simulink model "FSAC2021_V1_Running"  (R2014a)
settings: Solver=FixedStepDiscrete  StartTime=0.0  StopTime=inf  FixedStep=0.0005  RelTol=1e-3
model workspace (MAT data in the model file):
  AS_READY = Simulink.Parameter
  AS_READY.Value = 2
  AS_READY.DataType = 'uint8'
  AS_DRIVING = Simulink.Parameter
  AS_DRIVING.Value = 3
  AS_DRIVING.DataType = 'uint8'
  AS_OFF = Simulink.Parameter
  AS_OFF.Value = 1
  AS_OFF.DataType = 'uint8'
  AS_FINISH = Simulink.Parameter
  AS_FINISH.Value = 4
  AS_FINISH.DataType = 'uint8'
  AS_EMERGENCY = Simulink.Parameter
  AS_EMERGENCY.Value = 5
  AS_EMERGENCY.DataType = 'uint8'
  ENABLE = Simulink.Parameter
  ENABLE.Value = 1
  ENABLE.DataType = 'uint8'
  DISABLE = Simulink.Parameter
  DISABLE.Value = 0
  DISABLE.DataType = 'uint8'
  Tire_Radius = Simulink.Parameter
  Tire_Radius.Value = 234
  Tire_Radius.DataType = 'single'
  Ts = Simulink.Parameter
  Ts.Value = 0.0005
  Ts.DataType = 'double'
  Filter_Factor = Simulink.Parameter
  Filter_Factor.Value = 0.5
  Filter_Factor.DataType = 'single'
  Teeth_Wheel = Simulink.Parameter
  Teeth_Wheel.Value = 60
  Teeth_Wheel.DataType = 'uint8'
  BLINK = Simulink.Parameter
  BLINK.Value = 2
  BLINK.DataType = 'uint8'
  OFF = Simulink.Parameter
  OFF.Value = 0
  OFF.DataType = 'uint8'
  ON = Simulink.Parameter
  ON.Value = 1
  ON.DataType = 'uint8'
  EBS_DISABLE = Simulink.Parameter
  EBS_DISABLE.Value = 0
  EBS_DISABLE.DataType = 'uint8'
  EBS_ARMED = Simulink.Parameter
  EBS_ARMED.Value = 1
  EBS_ARMED.DataType = 'uint8'
  EBS_ENABLE = Simulink.Parameter
  EBS_ENABLE.Value = 2
  EBS_ENABLE.DataType = 'uint8'
  MANUAL_DRIVING = Simulink.Parameter
  MANUAL_DRIVING.Value = 6
  MANUAL_DRIVING.DataType = 'uint8'
  MANUAL_MODE = Simulink.Parameter
  MANUAL_MODE.Value = 6
  MANUAL_MODE.DataType = 'uint8'
  BUZZER_START = 1
  BUZZER_EBS = Simulink.Parameter
  BUZZER_EBS.Value = 2
  BUZZER_EBS.DataType = 'uint8'
  TRACKDRIVE = Simulink.Parameter
  TRACKDRIVE.Value = 3
  TRACKDRIVE.DataType = 'uint8'
  Self_Learn_Diff = Simulink.Parameter
  Self_Learn_Diff.Value = 150
  Self_Learn_Diff.DataType = 'uint16'
  Acc_Left_Full_mv = Simulink.Parameter
  Acc_Left_Full_mv.Value = 2000
  Acc_Left_Full_mv.DataType = 'single'
  Acc_Right_Full_mv = Simulink.Parameter
  Acc_Right_Full_mv.Value = 2000
  Acc_Right_Full_mv.DataType = 'single'
  Brk_Calib_Value = Simulink.Parameter
  Brk_Calib_Value.Value = 150
  Brk_Calib_Value.DataType = 'single'
  Brk_Use_Range = Simulink.Parameter
  Brk_Use_Range.Value = 1500
  Brk_Use_Range.DataType = 'single'
  Armed = Simulink.Parameter
  Armed.Value = 1
  Armed.DataType = 'uint8'
  Enable = Simulink.Parameter
  Enable.Value = 2
  Enable.DataType = 'uint8'
  Disable = Simulink.Parameter
  Disable.Value = 0
  Disable.DataType = 'uint8'
  High_V = Simulink.Parameter
  High_V.Value = 60
  High_V.DataType = 'uint8'
  reg_num = Simulink.Parameter
  reg_num.Value = 1
  reg_num.DataType = 'uint8'
  Acc_Diff = Simulink.Parameter
  Acc_Diff.Value = 0.3
  Acc_Diff.DataType = 'single'
  Mtr_Cabli = Simulink.Parameter
  Mtr_Cabli.Value = 3
  Mtr_Cabli.DataType = 'single'
  BMS_Cabli = Simulink.Parameter
  BMS_Cabli.Value = 3
  BMS_Cabli.DataType = 'single'
  EBS_Cabli = Simulink.Parameter
  EBS_Cabli.Value = 3.3
  EBS_Cabli.DataType = 'single'
  Acc_Right_Factor = Simulink.Parameter
  Acc_Right_Factor.Value = -0.0833
  Acc_Right_Factor.DataType = 'double'
  Acc_Left_Factor = Simulink.Parameter
  Acc_Left_Factor.Value = 0.045
  Acc_Left_Factor.DataType = 'double'
  Acc_Lft_Offset = Simulink.Parameter
  Acc_Lft_Offset.Value = -90
  Acc_Lft_Offset.DataType = 'int8'
  Acc_Right_Offset = Simulink.Parameter
  Acc_Right_Offset.Value = 408.33
  Acc_Right_Offset.DataType = 'single'
  RTeeth_Wheel = Simulink.Parameter
  RTeeth_Wheel.Value = 30
  RTeeth_Wheel.DataType = 'uint8'
  FTeeth_Wheel = Simulink.Parameter
  FTeeth_Wheel.Value = 60
  FTeeth_Wheel.DataType = 'uint8'
  Brk_Liquid_Prs_Offset = Simulink.Parameter
  Brk_Liquid_Prs_Offset.Value = 0
  Brk_Liquid_Prs_Offset.DataType = 'single'
  Brk_Liquid_Prs_Factor = Simulink.Parameter
  Brk_Liquid_Prs_Factor.Value = 0.001
  Brk_Liquid_Prs_Factor.DataType = 'double'
  EBS_Prs_Factor = Simulink.Parameter
  EBS_Prs_Factor.Value = 0.000303
  EBS_Prs_Factor.DataType = 'double'
  EBS_Prs_Offset = Simulink.Parameter
  EBS_Prs_Offset.Value = 0
  EBS_Prs_Offset.DataType = 'single'
  Mtr_Volt_Factor = Simulink.Parameter
  Mtr_Volt_Factor.Value = 33.33
  Mtr_Volt_Factor.DataType = 'single'
  Mtr_Volt_Offset = Simulink.Parameter
  Mtr_Volt_Offset.Value = 0
  Mtr_Volt_Offset.DataType = 'single'
  BMS_Output_Volt_Factor = Simulink.Parameter
  BMS_Output_Volt_Factor.Value = 33.33
  BMS_Output_Volt_Factor.DataType = 'single'
  BMS_Output_Volt_Offset = Simulink.Parameter
  BMS_Output_Volt_Offset.Value = 0
  BMS_Output_Volt_Offset.DataType = 'single'
  Min = Simulink.Parameter
  Min.Value = 10
  Min.DataType = 'uint8'
  ACC_LOCK_UPSET = Simulink.Parameter
  ACC_LOCK_UPSET.Value = 25
  ACC_LOCK_UPSET.DataType = 'uint8'
  BRK_DISPSENS_LOWLIMIT = Simulink.Parameter
  BRK_DISPSENS_LOWLIMIT.Value = 2
  BRK_DISPSENS_LOWLIMIT.DataType = 'single'
  BRK_ENGAGED = Simulink.Parameter
  BRK_ENGAGED.Value = 1
  BRK_ENGAGED.DataType = 'uint8'
  BRK_Engaged_Angle = Simulink.Parameter
  BRK_Engaged_Angle.Value = 10
  BRK_Engaged_Angle.DataType = 'int8'
  BRK_MOVE = Simulink.Parameter
  BRK_MOVE.Value = 3
  BRK_MOVE.DataType = 'uint8'
  BRK_MTR_RATIO = Simulink.Parameter
  BRK_MTR_RATIO.Value = 10
  BRK_MTR_RATIO.DataType = 'uint8'
  BRK_TOZERO = Simulink.Parameter
  BRK_TOZERO.Value = 2
  BRK_TOZERO.DataType = 'uint8'
  Brake = 11
  Brk_Pct2Angle = Simulink.Parameter
  Brk_Pct2Angle.Value = 0.9
  Brk_Pct2Angle.DataType = 'single'
  Brk_Prop2Angle = Simulink.Parameter
  Brk_Prop2Angle.Value = 1
  Brk_Prop2Angle.DataType = 'single'
  DIFF_RATIO = Simulink.Parameter
  DIFF_RATIO.Value = 5
  DIFF_RATIO.DataType = 'uint8'
  DISABLE1 = Simulink.Parameter
  DISABLE1.Value = 0
  DISABLE1.DataType = 'uint8'
  ENABLE1 = Simulink.Parameter
  ENABLE1.Value = 1
  ENABLE1.DataType = 'uint8'
  MANUAL_MODEL = Simulink.Parameter
  MANUAL_MODEL.Value = 6
  MANUAL_MODEL.DataType = 'uint8'
  PULSES_PER_CIRCLE = Simulink.Parameter
  PULSES_PER_CIRCLE.Value = 6400
  PULSES_PER_CIRCLE.DataType = 'auto'
  Pct2Kmh = Simulink.Parameter
  Pct2Kmh.Value = 0.2
  Pct2Kmh.DataType = 'double'
  Sensor_Acc_b = 101.85
  Sensor_Acc_k = -0.0185
  Str_Sen_Orig_Angle = -341
  TIRE_D = Simulink.Parameter
  TIRE_D.Value = 0.47
  TIRE_D.DataType = 'double'
  Tire_D = 0.47
  T = 0.05
libraries: simulink x402, ec55xxlib x134
(part 1 of 17)
settings Model: Creator=zxj  LastModifiedBy=zxj
settings OptimizationCC: InlineParams=on  InlineInvariantSignals=on  RollThreshold=9  StateBitsets=on  DataBitsets=on  UseTempVars=on  ZeroExternalMemoryAtStartup=off  ZeroInternalMemoryAtStartup=off  EfficientFloat2IntCast=on  OptimizeModelRefInitCode=on  LifeSpan=1
settings DebuggingCC: InheritedTsInSrcMsg=none  ParameterOverflowMsg=none
settings HardwareCC: ProdLargestAtomicInteger=Long  ProdLargestAtomicFloat=Double  ProdIntDivRoundTo=Zero  ProdEndianess=BigEndian  ProdHWDeviceType=Freescale MPC5500
settings RTWCC: SystemTargetFile=ec55xx.tlc  MakeCommand=make_rtw optimized_fixed_point=1  GenerateMakefile=off  TemplateMakefile=ec55xx_lcc.tmf  PostCodeGenCommand=ec55xx_pst_s2(buildInfo)  Description=Target for EC55XX  GenerateReport=on  ProcessScript=ec55xx_make_rtw_hook  IncludeHyperlinkInReport=on  LaunchReport=on
settings CodeAppCC: IgnoreCustomStorageClasses=off
settings STFCustomTargetCC: ModelReferenceCompliant=off  ConcurrentExecutionCompliant=off  IncludeMdlTerminateFcn=off  GeneratePreprocessorConditionals=Use local settings  CombineOutputUpdateFcns=on  SuppressErrorStatus=on  ERTCustomFileBanners=on  SupportContinuousTime=off  SupportNonInlinedSFcns=off  MATLABClassNameForMDSCustomization=Simulink.SoftwareTarget.ERTCustomization  GRTInterface=off  SystemTargetFile=ec55xx.tlc
settings ERTTargetCC: GenerateSampleERTMain=off  ModelReferenceCompliant=off  IncludeMdlTerminateFcn=off  SuppressErrorStatus=on  GenerateASAP2=on  ERTSrcFileBannerTemplate=ec55xx_code_template.cgt  ERTHdrFileBannerTemplate=ec55xx_code_template.cgt  ERTDataSrcFileTemplate=ec55xx_code_template.cgt  ERTDataHdrFileTemplate=ec55xx_code_template.cgt  ERTCustomFileTemplate=ec55xx_file_process.tlc

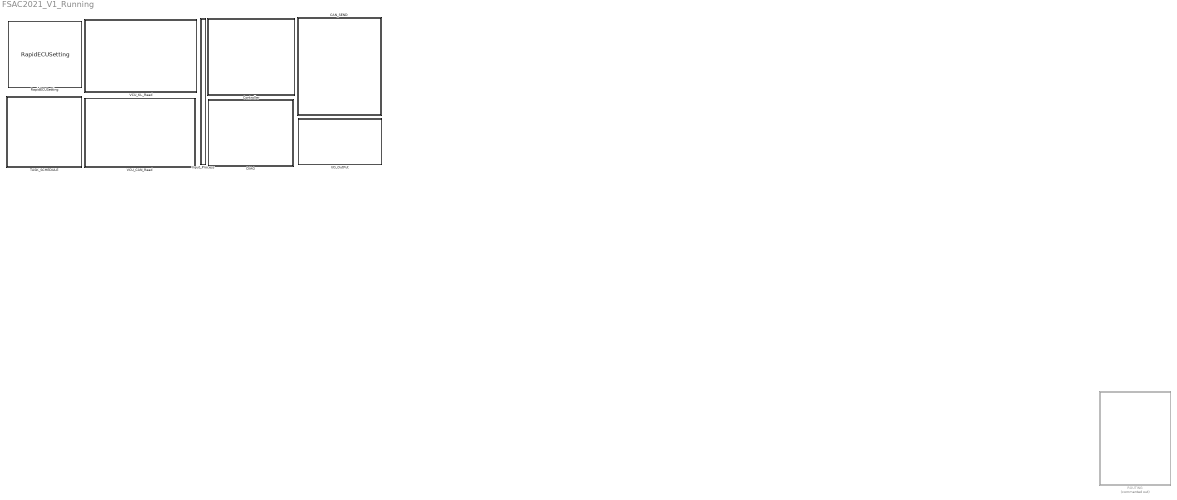
== system FSAC2021_V1_Running ==
  CAN_SEND : Subsystem
  Controller : Subsystem
  DIAG : Subsystem
  I/O_OutPut : Subsystem
  Input_Process : Subsystem
  ROUTING : Subsystem  Commented=on
  RapidECUSetting : ec55xxlib/RapidECU_U2/RapidECUSetting
      link override CAN: bcmt=Extended(29-bit ID)
      link override RTI: rtiperiod=0.0005
  TASK_SCHEDULE : Subsystem
  VCU_CAN_Read : Subsystem
  VCU_KL_Read : Subsystem

== system FSAC2021_V1_Running/CAN_SEND ==
  (BRK、STR、DRIVER) : Subsystem  SystemSampleTime=0.05
  From21 : From  Commented=on  GotoTag=Brk_Mtr_Enable_funCall  TagVisibility=global
  Rate Transition{1..19} (19 alike) : RateTransition  Deterministic=off
  Subsystem : Subsystem
  Subsystem1 : Subsystem
  Unit Delay{1..6} (6 alike) : UnitDelay  SampleTime=-1
  wires:
  [enable_operation_ctrl] -> Rate Transition4/1
  [new_set_pint_ctrl] -> Rate Transition5/1
  [abs_or_rel_ctrl] -> Rate Transition6/1
  [halt_ctrl] -> Rate Transition8/1
  [quick_stop_ctrl] -> Rate Transition3/1
  [enable_voltage_ctrl] -> Rate Transition2/1
  [position_set] -> Rate Transition9/1
  [switch_on_ctrl] -> Rate Transition1/1
  [nmt_nodeorder] -> Rate Transition11/1
  [nmt_nodectrl] -> Rate Transition12/1
  [encoder_msg_data] -> Rate Transition15/1
  [Brk_Mtr_GoalPos] -> Rate Transition17/1
  [Acc_Ctr] -> Rate Transition18/1
  Rate Transition17/1 -> Unit Delay3/1
  Rate Transition18/1 -> Unit Delay4/1
  Rate Transition10/1 -> Unit Delay5/1
  [BatVoltage_Out] -> Rate Transition10/1
  Rate Transition13/1 -> Unit Delay1/1
  Rate Transition14/1 -> Unit Delay2/1
  [Motor_Current_Speed] -> Rate Transition13/1
  [ASSI_State] -> Rate Transition14/1
  [Vel_Spd] -> Rate Transition16/1
  Rate Transition16/1 -> Unit Delay6/1
  [Fault_Reset] -> Rate Transition7/1
  Rate Transition7/1 -> Subsystem1/15(Fault_Reset)
  Rate Transition15/1 -> Subsystem1/14(Encoder_Msg_Data)
  [tmtsdocan] -> Subsystem1/13(Tmt_SDO_CAN_FunCall)
  [tmtnnmtcan] -> Subsystem1/10(Tmt_NMT_CAN_FunCall)
  Rate Transition11/1 -> Subsystem1/11(NMT_nodeorder)
  Rate Transition12/1 -> Subsystem1/12(NMT_nodectrl)
  [tmprdo1can] -> Subsystem1/1(Tmt_RPD01_CAN_FunCall)
  Rate Transition1/1 -> Subsystem1/2(Switch_On_Ctrl)
  Rate Transition6/1 -> Subsystem1/7(Abs_or_Rel_Ctrl)
  Rate Transition3/1 -> Subsystem1/4(Quick_Stop_Ctrl)
  Rate Transition2/1 -> Subsystem1/3(Enable_Voltage_Ctrl)
  Rate Transition4/1 -> Subsystem1/5(Enable_Operation_Ctrl)
  Rate Transition5/1 -> Subsystem1/6(New_Set_Point_Ctrl)
  Rate Transition8/1 -> Subsystem1/8(Halt_Ctrl)
  Rate Transition9/1 -> Subsystem1/9(Position_set)
  Unit Delay4/1 -> (BRK、STR、DRIVER)/2(Acc_Cmd)
  Unit Delay1/1 -> (BRK、STR、DRIVER)/4(Motor_Current_Speed)
  Unit Delay2/1 -> (BRK、STR、DRIVER)/5(ASSI_State)
  Unit Delay3/1 -> (BRK、STR、DRIVER)/1(Brk_Mtr_GoalPos)
  Unit Delay5/1 -> (BRK、STR、DRIVER)/3(BatVoltage_Out)
  Unit Delay6/1 -> (BRK、STR、DRIVER)/6(vspd)
  [ASSI_State] -> Rate Transition19/1
  Rate Transition19/1 -> Subsystem1/16(ASSI_STATE)

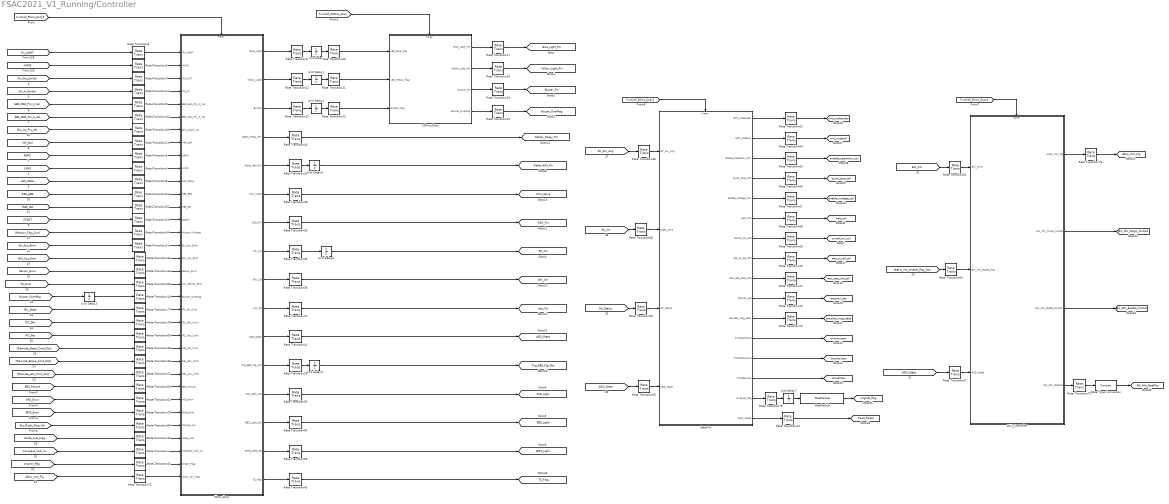
== system FSAC2021_V1_Running/Controller ==
  200ms_Duty : Subsystem
  50ms_Duty : Subsystem
  BCU_Controller : Subsystem
  Data Type Conversion : DataTypeConversion
  MeaModule : ec55xxlib/RapidECU_U2/11Calibration/MeaModule  signal=Steer_Origin_Flag
  Rate Transition{1..26,28..80} (79 alike) : RateTransition  Deterministic=off
  SteerCtr : Subsystem
  Unit Delay{,1..7} (8 alike) : UnitDelay  SampleTime=-1
  tag scope: ASSI_State=global, Acc_Ctr=global, Allow_Ctrl_Flg=global, BMS_Light=global, Blue_Light_Pin=global, Brk_Ctr=global, Brk_Mtr_Enable_funCall=global, Brk_Mtr_GoalPos=global, Brk_Mtr_Origin_funCall=global, Buzzer_Overflag=global, Buzzer_Pin=global, EBS_Light=global, Fault_Reset=global, IMD_Light=global, R2D_Pin=global, Relay_48V_Pin=global, Safety_Relay_Pin=global, Str_Ctr=global, TS_Flag=global, Trig_EBS_Flg_Out=global, VCU_Valve=global, Yellow_Light_Pin=global, abs_or_rel_ctrl=global, enable_operation_ctrl=global, enable_voltage_ctrl=global, encoder_msg_data=global, halt_ctrl=global, new_set_pint_ctrl=global, nmt_nodectrl=global, nmt_nodeorder=global, original_flag=global, position_set=global, quick_stop_ctrl=global, switch_on_ctrl=global, tmprdo1can=global, tmtnnmtcan=global, tmtsdocan=global
  wires:
  [On_Out_Switch] -> Rate Transition7/1
  [ASMS] -> Rate Transition5/1
  [AMI_State] -> Rate Transition8/1
  [EBS_GAS_Prs_2_Val] -> Rate Transition10/1
  [EBS_GAS_Prs_1_Val] -> Rate Transition9/1
  [HVMS] -> Rate Transition3/1
  Rate Transition8/1 -> 50ms_Duty/11(AMI_State)
  Rate Transition4/1 -> 50ms_Duty/10(LVMS)
  [LVMS] -> Rate Transition4/1
  Rate Transition10/1 -> 50ms_Duty/6(EBS_GAS_Prs_2_Val)
  Rate Transition7/1 -> 50ms_Duty/3(ON_OUT)
  [HV_LIGHT] -> Rate Transition2/1
  Rate Transition3/1 -> 50ms_Duty/2(HVMS)
  Rate Transition11/1 -> 50ms_Duty/8(Veh_Spd)
  Rate Transition2/1 -> 50ms_Duty/1(HV_LIGHT)
  [Vel_Spd] -> Rate Transition11/1
  Rate Transition9/1 -> 50ms_Duty/5(EBS_GAS_Prs_1_Val)
  Rate Transition5/1 -> 50ms_Duty/9(ASMS)
  [FunCall_50ms_Duty5] -> 50ms_Duty/Trigger
  [FunCall_200ms_Duty] -> 200ms_Duty/Trigger
  Rate Transition6/1 -> Unit Delay/1
  Rate Transition12/1 -> Unit Delay1/1
  Rate Transition13/1 -> Unit Delay2/1
  50ms_Duty/1(Blue_Light) -> Rate Transition6/1
  50ms_Duty/2(Yellow_Light) -> Rate Transition12/1
  50ms_Duty/3(Buzzer) -> Rate Transition13/1
  Unit Delay3/1 -> Rate Transition16/1
  Unit Delay/1 -> Rate Transition20/1
  Unit Delay1/1 -> Rate Transition21/1
  Unit Delay2/1 -> Rate Transition22/1
  [On_In_Switch] -> Rate Transition14/1
  Rate Transition14/1 -> 50ms_Duty/4(ON_IN)
  Rate Transition16/1 -> 50ms_Duty/20(Buzzer_Overflag)
  200ms_Duty/1(Blue_Light_Pin) -> Rate Transition17/1
  200ms_Duty/2(Yellow_Light_Pin) -> Rate Transition18/1
  200ms_Duty/3(Buzzer_Pin) -> Rate Transition19/1
  Rate Transition17/1 -> [Blue_Light_Pin]
  Rate Transition18/1 -> [Yellow_Light_Pin]
  Rate Transition19/1 -> [Buzzer_Pin]
  Rate Transition20/1 -> 200ms_Duty/1(LED_Blue_Flag)
  Rate Transition21/1 -> 200ms_Duty/2(LED_Yellow_Flag)
  Rate Transition22/1 -> 200ms_Duty/3(Buzzer_Flag)
  [START] -> Rate Transition23/1
  Rate Transition23/1 -> 50ms_Duty/14(START)
  [RES_EBS] -> Rate Transition24/1
  Rate Transition24/1 -> 50ms_Duty/12(RES_EBS)
  [RES_GO] -> Rate Transition25/1
  Rate Transition25/1 -> 50ms_Duty/13(RES_GO)
  Rate Transition26/1 -> 50ms_Duty/7(Brk_Liquid_Val)
  [Brs_Liq_Prs_Val] -> Rate Transition26/1
  200ms_Duty/4(Buzzer_Overflag) -> Rate Transition15/1
  Rate Transition15/1 -> [Buzzer_Overflag]
  [Buzzer_Overflag] -> Unit Delay3/1
  [Str_Sys_Error] -> Rate Transition31/1
  [Brk_Sys_Error] -> Rate Transition32/1
  [Sensor_Error] -> Rate Transition33/1
  Rate Transition31/1 -> 50ms_Duty/16(Str_Sys_Error)
  Rate Transition32/1 -> 50ms_Duty/17(Brk_Sys_Error)
  Rate Transition33/1 -> 50ms_Duty/18(Sensor_Error)
  [Mission_Flag_Out] -> Rate Transition34/1
  Rate Transition34/1 -> 50ms_Duty/15(Misson_Finished)
  50ms_Duty/8(Str_Ctr) -> Rate Transition35/1
  50ms_Duty/9(Brk_Ctr) -> Rate Transition36/1
  50ms_Duty/10(Acc_Ctr) -> Rate Transition37/1
  Rate Transition35/1 -> Unit Delay6/1
  Rate Transition36/1 -> [Brk_Ctr]
  Rate Transition37/1 -> [Acc_Ctr]
  Rate Transition38/1 -> [VCU_Valve]
  50ms_Duty/6(VCU_Valve) -> Rate Transition38/1
  Rate Transition39/1 -> [R2D_Pin]
  50ms_Duty/7(R2D_Pin) -> Rate Transition39/1
  50ms_Duty/4(Safety_Relay_Pin) -> Rate Transition40/1
  Rate Transition40/1 -> [Safety_Relay_Pin]
  50ms_Duty/11(ASSI_State) -> Rate Transition41/1
  Rate Transition41/1 -> [ASSI_State]
  [Node_Lost_Flag] -> Rate Transition42/1
  Rate Transition42/1 -> 50ms_Duty/31(Node_Lost)
  [Remote_Acc_Cmd_Out] -> Rate Transition47/1
  [Remote_Steer_Cmd_Out] -> Rate Transition49/1
  Rate Transition47/1 -> 50ms_Duty/26(Res_Acc_Cmd)
  [Remote_Brake_Cmd_Out] -> Rate Transition48/1
  Rate Transition49/1 -> 50ms_Duty/24(Res_Str_Cmd)
  Rate Transition48/1 -> 50ms_Duty/25(Res_Brk_Cmd)
  50ms_Duty/5(Relay_48V_Pin) -> Rate Transition30/1
  Rate Transition30/1 -> Unit Delay4/1
  Unit Delay4/1 -> [Relay_48V_Pin]
  [TS_Error] -> Rate Transition50/1
  Rate Transition50/1 -> 50ms_Duty/19(Acc_Sensor_Error)
  50ms_Duty/12(Trig_EBS_Flg_Out) -> Rate Transition28/1
  [EBS_Failure] -> Rate Transition51/1
  Rate Transition51/1 -> 50ms_Duty/27(EBS_Failure)
  Rate Transition28/1 -> Unit Delay5/1
  Unit Delay5/1 -> [Trig_EBS_Flg_Out]
  [BMS_Error] -> Rate Transition29/1
  Rate Transition29/1 -> 50ms_Duty/29(BMS_Error)
  Rate Transition52/1 -> 50ms_Duty/28(IMD_Error)
  [IMD_Error] -> Rate Transition52/1
  50ms_Duty/13(IMD_Light_Sts) -> Rate Transition53/1
  50ms_Duty/14(EBS_Light_Sts) -> Rate Transition54/1
  50ms_Duty/15(BMS_Light_Sts) -> Rate Transition55/1
  Rate Transition53/1 -> [IMD_Light]
  Rate Transition54/1 -> [EBS_Light]
  Rate Transition55/1 -> [BMS_Light]
  Rate Transition56/1 -> 50ms_Duty/30(Manual_Acc)
  [Acc_Right_Disp_Val] -> Rate Transition56/1
  SteerCtr/9(New_Set_Point_Ctrl) -> Rate Transition72/1
  SteerCtr/10(Position_set) -> Rate Transition73/1
  SteerCtr/11(Encoder_Msg_Data) -> Rate Transition74/1
  SteerCtr/2(NMT_nodectrl) -> Rate Transition64/1
  SteerCtr/3(Enable_Operation_Ctrl) -> Rate Transition65/1
  SteerCtr/4(Quick_Stop_Ctrl) -> Rate Transition66/1
  SteerCtr/5(Enable_Voltage_Ctrl) -> Rate Transition67/1
  SteerCtr/6(Halt_Ctrl) -> Rate Transition68/1
  SteerCtr/7(Switch_On_Ctrl) -> Rate Transition69/1
  SteerCtr/8(Abs_or_Rel_Ctrl) -> Rate Transition70/1
  SteerCtr/1(NMT_nodeorder) -> Rate Transition62/1
  [Str_Ctr] -> Rate Transition58/1
  [Str_Status] -> Rate Transition59/1
  [ASSI_State] -> Rate Transition60/1
  [Brk_Ctr] -> Rate Transition61/1
  [Brake_mtr_enable_flag_Out] -> Rate Transition63/1
  BCU_Controller/1(Allow_Ctrl_Flg) -> Rate Transition76/1
  BCU_Controller/4(Brk_Mtr_GoalPos) -> Rate Transition79/1
  Data Type Conversion/1 -> [Brk_Mtr_GoalPos]
  Rate Transition58/1 -> SteerCtr/2(Steer_Cmd)
  Rate Transition59/1 -> SteerCtr/3(Str_Status)
  Rate Transition60/1 -> SteerCtr/4(ASSI_State)
  Rate Transition61/1 -> BCU_Controller/1(Brk_Cmd)
  Rate Transition63/1 -> BCU_Controller/2(Brk_Mtr_Enable_Flg)
  Rate Transition62/1 -> [nmt_nodeorder]
  Rate Transition64/1 -> [nmt_nodectrl]
  Rate Transition65/1 -> [enable_operation_ctrl]
  Rate Transition66/1 -> [quick_stop_ctrl]
  Rate Transition67/1 -> [enable_voltage_ctrl]
  Rate Transition68/1 -> [halt_ctrl]
  Rate Transition69/1 -> [switch_on_ctrl]
  Rate Transition70/1 -> [abs_or_rel_ctrl]
  Rate Transition72/1 -> [new_set_pint_ctrl]
  Rate Transition73/1 -> [position_set]
  Rate Transition74/1 -> [encoder_msg_data]
  SteerCtr/15(Original_Flag) -> Rate Transition75/1
  Rate Transition76/1 -> [Allow_Ctrl_Flg]
  BCU_Controller/2(Brk_Mtr_Origin_funCall) -> [Brk_Mtr_Origin_funCall]
  BCU_Controller/3(Brk_Mtr_Enable_funCall) -> [Brk_Mtr_Enable_funCall]
  Rate Transition79/1 -> Data Type Conversion/1
  Rate Transition75/1 -> Unit Delay7/1
  SteerCtr/12(TmtNNMTCAN) -> [tmtnnmtcan]
  SteerCtr/13(TmtRPDO1CAN) -> [tmprdo1can]
  SteerCtr/14(TmtSDOCAN) -> [tmtsdocan]
  [FunCall_50ms_Duty1] -> SteerCtr/Trigger
  [FunCall_50ms_Duty3] -> BCU_Controller/Trigger
  Rate Transition1/1 -> 50ms_Duty/32(Compare_Volt_mv)
  [Compare_Volt_mv] -> Rate Transition1/1
  50ms_Duty/16(TS_Flag) -> Rate Transition43/1
  Rate Transition43/1 -> [TS_Flag]
  MeaModule/1 -> [original_flag]
  SteerCtr/16(Fault_Reset) -> Rate Transition44/1
  Rate Transition44/1 -> [Fault_Reset]
  Unit Delay6/1 -> [Str_Ctr]
  Rate Transition45/1 -> 50ms_Duty/33(Origin_Flag)
  [original_flag] -> Rate Transition45/1
  Unit Delay7/1 -> MeaModule/1
  [Str_Snr_Ang] -> Rate Transition46/1
  Rate Transition46/1 -> SteerCtr/1(Str_Snr_Ang)
  [ASSI_State] -> Rate Transition57/1
  Rate Transition57/1 -> BCU_Controller/3(ASSI_State)
  Rate Transition71/1 -> 50ms_Duty/34(Allow_Ctr_Flag)
  [Allow_Ctrl_Flg] -> Rate Transition71/1
  [IPC_Steer] -> Rate Transition77/1
  [IPC_Acc] -> Rate Transition80/1
  [IPC_Brk] -> Rate Transition78/1
  Rate Transition77/1 -> 50ms_Duty/21(IPC_Str_Cmd)
  Rate Transition78/1 -> 50ms_Duty/22(IPC_Brk_Cmd)
  Rate Transition80/1 -> 50ms_Duty/23(IPC_Acc_Cmd)

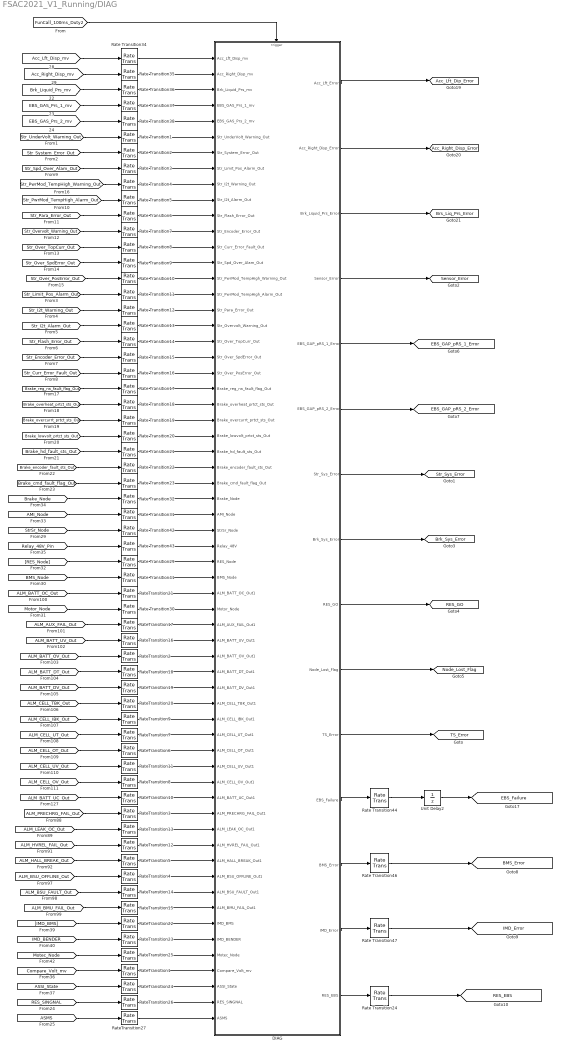
== system FSAC2021_V1_Running/DIAG ==
  DIAG : Subsystem
  Rate Transition{1..24,29..32,34..38,41..44,46..47} (39 alike) : RateTransition  Deterministic=off
  RateTransition{1..27} (27 alike) : RateTransition
  Unit Delay2 : UnitDelay  SampleTime=-1
  tag scope: Acc_Lft_Dip_Error=global, Acc_Right_Disp_Error=global, BMS_Error=global, Brk_Sys_Error=global, Brs_Liq_Prs_Error=global, EBS_Failure=global, EBS_GAP_pRS_1_Error=global, EBS_GAP_pRS_2_Error=global, IMD_Error=global, Node_Lost_Flag=global, RES_EBS=global, RES_GO=global, Sensor_Error=global, Str_Sys_Error=global, TS_Error=global
  wires:
  DIAG/1(Acc_Lft_Error) -> [Acc_Lft_Dip_Error]
  Rate Transition36/1 -> DIAG/3(Brk_Liquid_Prs_mv)
  DIAG/2(Acc_Right_Disp_Error) -> [Acc_Right_Disp_Error]
  DIAG/3(Brk_Liquid_Prs_Error) -> [Brs_Liq_Prs_Error]
  Rate Transition35/1 -> DIAG/2(Acc_Right_Disp_mv)
  Rate Transition37/1 -> DIAG/4(EBS_GAS_Prs_1_mv)
  Rate Transition38/1 -> DIAG/5(EBS_GAS_Prs_2_mv)
  Rate Transition34/1 -> DIAG/1(Acc_Lft_Disp_mv)
  [Brk_Liquid_Prs_mv] -> Rate Transition36/1
  [Acc_Lft_Disp_mv] -> Rate Transition34/1
  [EBS_GAS_Prs_1_mv] -> Rate Transition37/1
  [EBS_GAS_Prs_2_mv] -> Rate Transition38/1
  [Acc_Right_Disp_mv] -> Rate Transition35/1
  [FunCall_100ms_Duty2] -> DIAG/Trigger
  [Str_UnderVolt_Warning_Out] -> Rate Transition1/1
  [Str_System_Error_Out] -> Rate Transition2/1
  [Str_Spd_Over_Alam_Out] -> Rate Transition3/1
  [Str_PwrMod_TempHigh_Warning_Out] -> Rate Transition4/1
  [Str_PwrMod_TempHigh_Alarm_Out] -> Rate Transition5/1
  [Str_Para_Error_Out] -> Rate Transition6/1
  [Str_Overvolt_Warning_Out] -> Rate Transition7/1
  [Str_Over_TopCurr_Out] -> Rate Transition8/1
  [Str_Over_SpdError_Out] -> Rate Transition9/1
  [Str_Over_PosError_Out] -> Rate Transition10/1
  [Str_Limit_Pos_Alarm_Out] -> Rate Transition11/1
  [Str_I2t_Warning_Out] -> Rate Transition12/1
  [Str_I2t_Alarm_Out] -> Rate Transition13/1
  [Str_Flash_Error_Out] -> Rate Transition14/1
  [Str_Encoder_Error_Out] -> Rate Transition15/1
  [Str_Curr_Error_Fault_Out] -> Rate Transition16/1
  Rate Transition1/1 -> DIAG/6(Str_UnderVolt_Warning_Out)
  Rate Transition2/1 -> DIAG/7(Str_System_Error_Out)
  Rate Transition3/1 -> DIAG/8(Str_Limit_Pos_Alarm_Out)
  Rate Transition4/1 -> DIAG/9(Str_I2t_Warning_Out)
  Rate Transition5/1 -> DIAG/10(Str_I2t_Alarm_Out)
  Rate Transition6/1 -> DIAG/11(Str_Flash_Error_Out)
  Rate Transition7/1 -> DIAG/12(Str_Encoder_Error_Out)
  Rate Transition8/1 -> DIAG/13(Str_Curr_Error_Fault_Out)
  Rate Transition9/1 -> DIAG/14(Str_Spd_Over_Alam_Out)
  Rate Transition10/1 -> DIAG/15(Str_PwrMod_TempHigh_Warning_Out)
  Rate Transition11/1 -> DIAG/16(Str_PwrMod_TempHigh_Alarm_Out)
  Rate Transition12/1 -> DIAG/17(Str_Para_Error_Out)
  Rate Transition13/1 -> DIAG/18(Str_Overvolt_Warning_Out)
  Rate Transition15/1 -> DIAG/20(Str_Over_SpdError_Out)
  Rate Transition14/1 -> DIAG/19(Str_Over_TopCurr_Out)
  Rate Transition16/1 -> DIAG/21(Str_Over_PosError_Out)
  DIAG/4(Sensor_Error) -> [Sensor_Error]
  DIAG/7(Str_Sys_Error) -> [Str_Sys_Error]
  [Brake_overcurrt_prtct_sts_Out] -> Rate Transition19/1
  [Brake_overheat_prtct_sts_Out] -> Rate Transition18/1
  [Brake_reg_rw_fault_flag_Out] -> Rate Transition17/1
  [Brake_cmd_fault_flag_Out] -> Rate Transition23/1
  [Brake_hd_fault_sts_Out] -> Rate Transition21/1
  [Brake_encoder_fault_sts_Out] -> Rate Transition22/1
  [Brake_lowvolt_prtct_sts_Out] -> Rate Transition20/1
  Rate Transition17/1 -> DIAG/22(Brake_reg_rw_fault_flag_Out)
  Rate Transition18/1 -> DIAG/23(Brake_overheat_prtct_sts_Out)
  Rate Transition19/1 -> DIAG/24(Brake_overcurrt_prtct_sts_Out)
  Rate Transition20/1 -> DIAG/25(Brake_lowvolt_prtct_sts_Out)
  Rate Transition21/1 -> DIAG/26(Brake_hd_fault_sts_Out)
  Rate Transition22/1 -> DIAG/27(Brake_encoder_fault_sts_Out)
  Rate Transition23/1 -> DIAG/28(Brake_cmd_fault_flag_Out)
  DIAG/8(Brk_Sys_Error) -> [Brk_Sys_Error]
  DIAG/9(RES_GO) -> [RES_GO]
  [RES_Node] -> Rate Transition29/1
  [Motor_Node] -> Rate Transition30/1
  [AMI_Node] -> Rate Transition31/1
  [Brake_Node] -> Rate Transition32/1
  [BMS_Node] -> Rate Transition41/1
  [StrSr_Node] -> Rate Transition42/1
  Rate Transition29/1 -> DIAG/33(RES_Node)
  Rate Transition30/1 -> DIAG/36(Motor_Node)
  Rate Transition31/1 -> DIAG/30(AMI_Node)
  Rate Transition32/1 -> DIAG/29(Brake_Node)
  Rate Transition41/1 -> DIAG/34(BMS_Node)
  Rate Transition42/1 -> DIAG/31(StrSr_Node)
  DIAG/10(Node_Lost_Flag) -> [Node_Lost_Flag]
  [Relay_48V_Pin] -> Rate Transition43/1
  Rate Transition43/1 -> DIAG/32(Relay_48V)
  DIAG/11(TS_Error) -> [TS_Error]
  DIAG/5(EBS_GAP_pRS_1_Error) -> [EBS_GAP_pRS_1_Error]
  DIAG/12(EBS_Failure) -> Rate Transition44/1
  Rate Transition44/1 -> Unit Delay2/1
  Unit Delay2/1 -> [EBS_Failure]
  DIAG/6(EBS_GAP_pRS_2_Error) -> [EBS_GAP_pRS_2_Error]
  [ALM_BATT_OV_Out] -> RateTransition2/1
  RateTransition2/1 -> DIAG/39(ALM_BATT_OV_Out1)
  [ALM_PRECHRG_FAIL_Out] -> RateTransition3/1
  RateTransition3/1 -> DIAG/49(ALM_PRECHRG_FAIL_Out1)
  [ALM_BSU_OFFLINE_Out] -> RateTransition4/1
  RateTransition4/1 -> DIAG/53(ALM_BSU_OFFLINE_Out1)
  [ALM_HALL_BREAK_Out] -> RateTransition5/1
  RateTransition5/1 -> DIAG/52(ALM_HALL_BREAK_Out1)
  [ALM_CELL_OT_Out] -> RateTransition6/1
  RateTransition6/1 -> DIAG/45(ALM_CELL_OT_Out1)
  [ALM_CELL_UT_Out] -> RateTransition7/1
  RateTransition7/1 -> DIAG/44(ALM_CELL_UT_Out1)
  [ALM_CELL_OV_Out] -> RateTransition8/1
  RateTransition8/1 -> DIAG/47(ALM_CELL_OV_Out1)
  [ALM_CELL_IBK_Out] -> RateTransition9/1
  RateTransition9/1 -> DIAG/43(ALM_CELL_IBK_Out1)
  [ALM_BATT_UC_Out] -> RateTransition10/1
  RateTransition10/1 -> DIAG/48(ALM_BATT_UC_Out1)
  [ALM_CELL_UV_Out] -> RateTransition11/1
  RateTransition11/1 -> DIAG/46(ALM_CELL_UV_Out1)
  [ALM_HVREL_FAIL_Out] -> RateTransition12/1
  RateTransition12/1 -> DIAG/51(ALM_HVREL_FAIL_Out1)
  [ALM_LEAK_OC_Out] -> RateTransition13/1
  RateTransition13/1 -> DIAG/50(ALM_LEAK_OC_Out1)
  [ALM_BSU_FAULT_Out] -> RateTransition14/1
  RateTransition14/1 -> DIAG/54(ALM_BSU_FAULT_Out1)
  [ALM_BMU_FAIL_Out] -> RateTransition15/1
  RateTransition15/1 -> DIAG/55(ALM_BMU_FAIL_Out1)
  [ALM_BATT_UV_Out] -> RateTransition16/1
  RateTransition16/1 -> DIAG/38(ALM_BATT_UV_Out1)
  [ALM_AUX_FAIL_Out] -> RateTransition17/1
  RateTransition17/1 -> DIAG/37(ALM_AUX_FAIL_Out1)
  [ALM_BATT_DT_Out] -> RateTransition18/1
  RateTransition18/1 -> DIAG/40(ALM_BATT_DT_Out1)
  [ALM_BATT_DV_Out] -> RateTransition19/1
  RateTransition19/1 -> DIAG/41(ALM_BATT_DV_Out1)
  [ALM_CELL_TBK_Out] -> RateTransition20/1
  RateTransition20/1 -> DIAG/42(ALM_CELL_TBK_Out1)
  [ALM_BATT_OC_Out] -> RateTransition21/1
  RateTransition21/1 -> DIAG/35(ALM_BATT_OC_Out1)
  DIAG/13("BMS_Error ") -> Rate Transition46/1
  Rate Transition46/1 -> [BMS_Error]
  [IMD_BMS] -> RateTransition22/1
  [IMD_BENDER] -> RateTransition23/1
  RateTransition22/1 -> DIAG/56("IMD_BMS ")
  RateTransition23/1 -> DIAG/57("IMD_BENDER ")
  DIAG/14(IMD_Error) -> Rate Transition47/1
  Rate Transition47/1 -> [IMD_Error]
  RateTransition25/1 -> DIAG/58(Motec_Node)
  [Motec_Node] -> RateTransition25/1
  RateTransition1/1 -> DIAG/59(Compare_Volt_mv)
  [Compare_Volt_mv] -> RateTransition1/1
  RateTransition24/1 -> DIAG/60(ASSI_State)
  [ASSI_State] -> RateTransition24/1
  [RES_SINGNAL] -> RateTransition26/1
  RateTransition26/1 -> DIAG/61(RES_SINGNAL)
  [ASMS] -> RateTransition27/1
  RateTransition27/1 -> DIAG/62(ASMS)
  DIAG/15(RES_EBS) -> Rate Transition24/1
  Rate Transition24/1 -> [RES_EBS]

== system FSAC2021_V1_Running/I//O_OutPut ==
  Subsystem : Subsystem
  wires:
  [Blue_Light_Pin] -> Subsystem/1(Blue_Light_Pin)
  [Yellow_Light_Pin] -> Subsystem/2(Yellow_Light_Pin)
  [Buzzer_Pin] -> Subsystem/3(Buzzer_pin)
  [Safety_Relay_Pin] -> Subsystem/4(Safety_Relay_Pin)
  [Relay_48V_Pin] -> Subsystem/5(Relay_48V_Pin)
  [R2D_Pin] -> Subsystem/6(R2D_pin)
  [VCU_Valve] -> Subsystem/7(VCU_valve)
  [IMD_Light] -> Subsystem/8(IMD_Light)
  [EBS_Light] -> Subsystem/9(EBS_Light)
  [BMS_Light] -> Subsystem/10(BMS_Light)
  [FunCall_50ms_Duty10] -> Subsystem/Trigger

== system FSAC2021_V1_Running/Input_Process ==
  KL_Sig_Process : Subsystem
  Rate Transition{3..7,9..12,14..15,18..19,21..26} (19 alike) : RateTransition  Deterministic=off
  tag scope: Acc_Lft_Dip_Val=global, Acc_Right_Disp_Val=global, Brs_Liq_Prs_Val=global, EBS_GAS_Prs_1_Val=global, EBS_GAS_Prs_2_Val=global, Vel_Spd=global, Whl_Spd_FF_Val=global, Whl_Spd_FL_Val=global, Whl_Spd_RL_Val=global, Whl_Spd_RR_Val=global
  wires:
  [Acc_Lft_Disp_mv] -> Rate Transition21/1
  [EBS_GAS_Prs_1_mv] -> Rate Transition14/1
  [EBS_GAS_Prs_2_mv] -> Rate Transition24/1
  [Brk_Liquid_Prs_mv] -> Rate Transition23/1
  [Acc_Right_Disp_mv] -> Rate Transition22/1
  KL_Sig_Process/1(Vel_Spd) -> Rate Transition15/1
  KL_Sig_Process/4(Whl_Spd_RL_Val) -> Rate Transition10/1
  KL_Sig_Process/2(Whl_Spd_FL_Val) -> Rate Transition12/1
  KL_Sig_Process/3(Whl_Spd_FF_Val) -> Rate Transition11/1
  Rate Transition19/1 -> KL_Sig_Process/2(FR_WhlSpd_Hz)
  KL_Sig_Process/5(Whl_Spd_RR_Val) -> Rate Transition9/1
  Rate Transition26/1 -> KL_Sig_Process/4(RR_WhlSpd_Hz)
  [RR_WhlSpd_Hz] -> Rate Transition26/1
  Rate Transition25/1 -> KL_Sig_Process/3(RL_WhlSpd_Hz)
  Rate Transition18/1 -> KL_Sig_Process/1(FL_WhlSpd_Hz)
  [RL_WhlSpd_Hz] -> Rate Transition25/1
  [FL_WhlSpd_Hz] -> Rate Transition18/1
  [FR_WhlSpd_Hz] -> Rate Transition19/1
  KL_Sig_Process/7(Acc_Right_Disp_Val) -> Rate Transition6/1
  KL_Sig_Process/6(Acc_Lft_Disp_Val) -> Rate Transition7/1
  Rate Transition24/1 -> KL_Sig_Process/9(EBS_GAS_Prs_2_mv)
  Rate Transition23/1 -> KL_Sig_Process/7(Brk_Liquid_Prs_mv)
  KL_Sig_Process/10(EBS_GAS_Prs_2_Val) -> Rate Transition3/1
  Rate Transition21/1 -> KL_Sig_Process/5(Acc_Lft_Disp_mv)
  KL_Sig_Process/8(Brk_Liquid_Prs_Val) -> Rate Transition5/1
  Rate Transition22/1 -> KL_Sig_Process/6(Acc_Right_Disp_mv)
  KL_Sig_Process/9(EBS_GAS_Prs_1_Val) -> Rate Transition4/1
  Rate Transition14/1 -> KL_Sig_Process/8(EBS_GAS_Prs_1_mv)
  [FunCall_20ms_Duty] -> KL_Sig_Process/Trigger
  Rate Transition3/1 -> [EBS_GAS_Prs_2_Val]
  Rate Transition4/1 -> [EBS_GAS_Prs_1_Val]
  Rate Transition5/1 -> [Brs_Liq_Prs_Val]
  Rate Transition6/1 -> [Acc_Right_Disp_Val]
  Rate Transition7/1 -> [Acc_Lft_Dip_Val]
  Rate Transition9/1 -> [Whl_Spd_RR_Val]
  Rate Transition10/1 -> [Whl_Spd_RL_Val]
  Rate Transition11/1 -> [Whl_Spd_FF_Val]
  Rate Transition12/1 -> [Whl_Spd_FL_Val]
  Rate Transition15/1 -> [Vel_Spd]

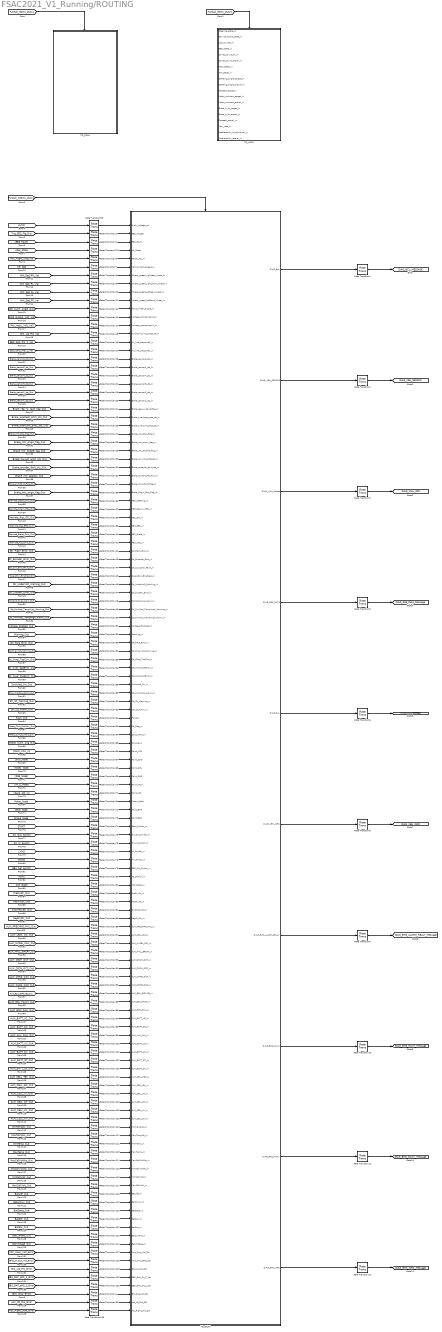
== system FSAC2021_V1_Running/ROUTING ==
  Rate Transition{1..4,6..130} (129 alike) : RateTransition  Deterministic=off
  Rate Transtion{1..3,5..6,8..12,33,131} (12 alike) : RateTransition  Deterministic=off
  TO_ACAN : Subsystem
  TO_DCAN : Subsystem
  TO_PCAN : Subsystem
  tag scope: DIAG_BCU_MESSAGE=global, DIAG_BMS_ALARM_RELAY_Message=global, DIAG_BMS_INFO_Message=global, DIAG_BMS_MAXT_Message=global, DIAG_BMS_MAXV_Message=global, DIAG_RES_Data_Message=global, DIAG_SCU_Message=global, DIAG_VEH_INFO=global, DIAG_VEH_SENSOR=global, DIAG_WHL_SPD=global
  wires:
  [FunCall_50ms_Duty4] -> TO_PCAN/Trigger
  [FunCall_50ms_Duty3] -> TO_ACAN/Trigger
  [Trig_EBS_Flg_Out] -> Rate Transition1/1
  [Whl_Spd_RL_Val] -> Rate Transition9/1
  [Brake_reg_rw_fault_flag_Out] -> Rate Transition24/1
  [BMS_Output_Volt_Val] -> Rate Transition13/1
  [Vel_Spd] -> Rate Transition7/1
  [Mtr_Input_Volt_Val] -> Rate Transition14/1
  [Brake_mtr_enable_flag_Out] -> Rate Transition29/1
  [EBS_GAS_Prs_1_Val] -> Rate Transition17/1
  [Brake_mtr_origin_flag_Out] -> Rate Transition28/1
  [Brake_encoder_fault_sts_Out] -> Rate Transition31/1
  [Whl_Spd_FL_Val] -> Rate Transition10/1
  [Brake_sensor5_sts_Out] -> Rate Transition20/1
  [Str_Currt_Angle_Out] -> Rate Transition12/1
  [EBS_Fault] -> Rate Transition2/1
  [Whl_Spd_FF_Val] -> Rate Transition11/1
  [Whl_Spd_RR_Val] -> Rate Transition8/1
  [Brake_overcurrt_prtct_sts_Out] -> Rate Transition26/1
  [Brake_lowvolt_prtct_sts_Out] -> Rate Transition30/1
  [Brake_sensor3_sts_Out] -> Rate Transition22/1
  [Str_Flash_Error_Out] -> Rate Transition42/1
  [Str_Over_PosError_Out] -> Rate Transition57/1
  [Str_Encoder_Error_Out] -> Rate Transition43/1
  [Motec_Currt_Current_Out] -> Rate Transition64/1
  [Str_PwrMod_TempHigh_Alarm_Out] -> Rate Transition50/1
  [Brake_mtr_stop_flag_Out] -> Rate Transition27/1
  [EBS_GAS_Prs_2_Val] -> Rate Transition16/1
  [Brake_mtr_goalpos_Out] -> Rate Transition32/1
  [Remote_Brake_Cmd_Out] -> Rate Transition40/1
  [Remote_Res_EBS_Out] -> Rate Transition38/1
  [Point_VCU_in] -> Rate Transition66/1
  [Brake_sensor1_sts_Out] -> Rate Transition23/1
  [Brake_sensor6_sts_Out] -> Rate Transition18/1
  [Str_Curr_Error_Fault_Out] -> Rate Transition44/1
  [Brake_sensor4_sts_Out] -> Rate Transition21/1
  [Str_System_Error_Out] -> Rate Transition47/1
  [Remote_Res_GO_Out] -> Rate Transition39/1
  [Fault_Out] -> Rate Transition62/1
  [Remote_Acc_Cmd_Out] -> Rate Transition41/1
  [Brs_Liq_Prs_Val] -> Rate Transition15/1
  [Operation_Enabled_Out] -> Rate Transition45/1
  [Remote_Steer_Cmd_Out] -> Rate Transition36/1
  [Remote_Origin_Flag_Out] -> Rate Transition37/1
  [Brake_sensor2_sts_Out] -> Rate Transition19/1
  [Brake_cmd_fault_flag_Out] -> Rate Transition34/1
  [Str_Spd_Over_Alam_Out] -> Rate Transition48/1
  [Str_I2t_Alarm_Out] -> Rate Transition61/1
  [Str_PwrMod_TempHigh_Warning_Out] -> Rate Transition49/1
  [Str_UnderVolt_Warning_Out] -> Rate Transition46/1
  [Str_Para_Error_Out] -> Rate Transition53/1
  [Voltage_Enabled_Out] -> Rate Transition51/1
  [Brake_mtr_origin_flag_Out] -> Rate Transition35/1
  [ALM_HALL_BREAK_Out] -> Rate Transition89/1
  [PreRlyStr_Out] -> Rate Transition82/1
  [MCU_Node] -> Rate Transition70/1
  [EBS_Rel_Switch] -> Rate Transition79/1
  [HVMS] -> Rate Transition78/1
  [ALM_CHRG_OCT_Out] -> Rate Transition92/1
  [StrSr_Node] -> Rate Transition67/1
  [RES_Node] -> Rate Transition69/1
  [ALM_CHRG_OCS_Out] -> Rate Transition93/1
  [OnChrRlyStr_Out] -> Rate Transition84/1
  [ALM_BMU_FAIL_Out] -> Rate Transition96/1
  [Motec_Node] -> Rate Transition68/1
  [Str_Over_SpdError_Out] -> Rate Transition56/1
  [PosRlyStr_Out] -> Rate Transition83/1
  [Point_IPC_in] -> Rate Transition71/1
  [ALM_DSCH_OCS_Out] -> Rate Transition91/1
  [BMS_Node] -> Rate Transition72/1
  [Str_Over_TopCurr_Out] -> Rate Transition55/1
  [Swtiched_On_Out] -> Rate Transition58/1
  [Str_I2t_Warning_Out] -> Rate Transition60/1
  [START] -> Rate Transition74/1
  [Str_Limit_Pos_Alarm_Out] -> Rate Transition59/1
  [AMI_State] -> Rate Transition81/1
  [Brake_Node] -> Rate Transition73/1
  [Str_Overvolt_Warning_Out] -> Rate Transition54/1
  [On_Out_Switch] -> Rate Transition75/1
  [On_In_Switch] -> Rate Transition76/1
  [ALM_PRECHRG_FAIL_Out] -> Rate Transition86/1
  [Warning_Out] -> Rate Transition52/1
  [LVMS] -> Rate Transition77/1
  [ASMS] -> Rate Transition80/1
  [ALM_BATT_OC_Out] -> Rate Transition98/1
  [ALM_CELL_TBK_Out] -> Rate Transition104/1
  [ALM_HVREL_FAIL_Out] -> Rate Transition88/1
  [ALM_BSU_OFFLINE_Out] -> Rate Transition94/1
  [ALM_CELL_OT_Out] -> Rate Transition107/1
  [MaxTempNo_Out] -> Rate Transition111/1
  [MinTemp_Out] -> Rate Transition112/1
  [ALM_BATT_DT_Out] -> Rate Transition102/1
  [ALM_LEAK_OC_Out] -> Rate Transition87/1
  [ALM_CELL_UT_Out] -> Rate Transition106/1
  [ALM_CELL_UV_Out] -> Rate Transition108/1
  [BatCurrent_Out] -> Rate Transition123/1
  [ALM_DSCH_OCT_Out] -> Rate Transition90/1
  [MaxTemp_Out] -> Rate Transition113/1
  [ALM_CELL_OV_Out] -> Rate Transition109/1
  Rate Transition1/1 -> TO_DCAN/2(EBS_Trigger)
  Rate Transition2/1 -> TO_DCAN/3(EBS_Fault)
  [ALM_CELL_IBK_Out] -> Rate Transition105/1
  [BatState_Out] -> Rate Transition120/1
  [MaxCellVolt_Out] -> Rate Transition117/1
  [ALM_BSU_FAULT_Out] -> Rate Transition95/1
  [MinTempNo_Out] -> Rate Transition110/1
  [ALM_BATT_DV_Out] -> Rate Transition103/1
  [BatSoc_Out] -> Rate Transition122/1
  [ALM_AUX_FAIL_Out] -> Rate Transition99/1
  [HVMS] -> Rate Transtion33/1
  [ALM_BATT_OV_Out] -> Rate Transition101/1
  [ASSI_State] -> Rate Transtion131/1
  [MinCellVoltNo_Out] -> Rate Transition115/1
  [ALM_BATT_UC_Out] -> Rate Transition97/1
  [ALM_BATT_UV_Out] -> Rate Transition100/1
  [NegRlyStr_Out] -> Rate Transition85/1
  [MaxCellVoltNo_Out] -> Rate Transition114/1
  Rate Transition11/1 -> TO_DCAN/10(Wheel_speed_leftfront_wheel_in)
  Rate Transition8/1 -> TO_DCAN/7(Wheel_speed_rightrear_whee_in)
  Rate Transition17/1 -> TO_DCAN/16(Air_line_pressure1_in)
  Rate Transition34/1 -> TO_DCAN/32(Brake_cmd_fault_flag_in)
  Rate Transition24/1 -> TO_DCAN/23(Brake_reg_rw_fault_flag_in)
  Rate Transition9/1 -> TO_DCAN/8(Wheel_speed_right_front_wheel_in)
  Rate Transition35/1 -> TO_DCAN/33(Brake_0rigin_End_flag_in)
  Rate Transition23/1 -> TO_DCAN/22(Brake_sensor1_sts_in)
  Rate Transition27/1 -> TO_DCAN/26(Brake_mtr_stop_flag_in)
  Rate Transition30/1 -> TO_DCAN/29(Brake_lowvolt_prtct_sts_in)
  [BatSoh_Out] -> Rate Transition121/1
  [BatVoltage_Out] -> Rate Transition124/1
  Rate Transition7/1 -> TO_DCAN/6(Veh_Current_Speed_in)
  Rate Transition14/1 -> TO_DCAN/13(Voltage_comparison1_in)
  Rate Transition26/1 -> TO_DCAN/25(Brake_overcurrt_prtct_sts_in)
  [Motec_Currt_Position_Out] -> Rate Transition63/1
  Rate Transition18/1 -> TO_DCAN/17(Brake_sensor6_sts_in)
  Rate Transition16/1 -> TO_DCAN/15(Air_line_pressure2_in)
  Rate Transition15/1 -> TO_DCAN/14(Hydraulic_line_pressure_in)
  Rate Transition20/1 -> TO_DCAN/18(Brake_sensor5_sts_in)
  Rate Transition6/1 -> TO_DCAN/5(Pedal_Acc_in)
  Rate Transition13/1 -> TO_DCAN/12(Voltage_comparison2_in)
  Rate Transition32/1 -> TO_DCAN/31(Brake_Current_Position_in)
  [Brake_overheat_prtct_sts_Out] -> Rate Transition25/1
  [BatAlmLv_Out] -> Rate Transition119/1
  [MinCellVolt_Out] -> Rate Transition116/1
  [BatLife_Out] -> Rate Transition118/1
  [Motec_Currt_Ang_Out] -> Rate Transition65/1
  Rate Transition12/1 -> TO_DCAN/11(Front_wheel_angle_in)
  Rate Transition10/1 -> TO_DCAN/9(Wheel_speed_leftrear_wheel_in)
  Rate Transition48/1 -> TO_DCAN/46(Str_Spd_Over_Alam_in)
  Rate Transition22/1 -> TO_DCAN/20(Brake_sensor3_sts_in)
  Rate Transition28/1 -> TO_DCAN/27(Brake_mtr_origin_flag_in)
  Rate Transition37/1 -> TO_DCAN/35(RES_Return_INFO_in)
  Rate Transition46/1 -> TO_DCAN/44(Str_UnderVolt_Warning_in)
  Rate Transition51/1 -> TO_DCAN/49(Voltage_Enabled_in)
  Rate Transition66/1 -> TO_DCAN/64(Point_VCU)
  Rate Transition40/1 -> TO_DCAN/38(RES_Brake_in)
  Rate Transition29/1 -> TO_DCAN/28(Brake_mtr_enable_flag_in)
  Rate Transition65/1 -> TO_DCAN/63(Str_Ang_in)
  Rate Transition41/1 -> TO_DCAN/39(RES_ACC_in)
  Rate Transition45/1 -> TO_DCAN/43(Operation_Enabled_in)
  Rate Transition44/1 -> TO_DCAN/42(Str_Curr_Error_Fault_in)
  Rate Transition62/1 -> TO_DCAN/60(Fault_in)
  Rate Transition21/1 -> TO_DCAN/19(Brake_sensor4_sts_in)
  Rate Transition42/1 -> TO_DCAN/40(Str_Flash_Error_in)
  Rate Transition53/1 -> TO_DCAN/51(Str_Para_Error_in)
  Rate Transition59/1 -> TO_DCAN/57(Str_Limit_Pos_Alarm_in)
  Rate Transition47/1 -> TO_DCAN/45(Str_System_Error_in)
  Rate Transition39/1 -> TO_DCAN/36(RES_GO_in)
  Rate Transition49/1 -> TO_DCAN/47(Str_PwrMod_TempHigh_Warning_in)
  Rate Transition61/1 -> TO_DCAN/59(Str_I2t_Alarm_in)
  Rate Transition67/1 -> TO_DCAN/65(Point_StrSr)
  Rate Transition36/1 -> TO_DCAN/34(RES_Steering_in)
  Rate Transition43/1 -> TO_DCAN/41(Str_Encoder_Error_in)
  Rate Transition64/1 -> TO_DCAN/62(Str_Current_in)
  Rate Transition50/1 -> TO_DCAN/48(Str_PwrMod_TempHigh_Alarm_in)
  Rate Transition31/1 -> TO_DCAN/30(Brake_encoder_fault_sts_in)
  Rate Transition52/1 -> TO_DCAN/50(Warning_in)
  Rate Transition38/1 -> TO_DCAN/37(RES_EBS_in)
  Rate Transition19/1 -> TO_DCAN/21(Brake_sensor2_sts_in)
  Rate Transition25/1 -> TO_DCAN/24(Brake_overheat_prtct_sts_in)
  Rate Transition73/1 -> TO_DCAN/72(Point_BCU)
  Rate Transition68/1 -> TO_DCAN/66(Point_SCU)
  Rate Transition85/1 -> TO_DCAN/84(NegRlyStr_in)
  Rate Transition93/1 -> TO_DCAN/92(ALM_CHRG_OCS_in)
  Rate Transition69/1 -> TO_DCAN/67(Point_RES)
  Rate Transition90/1 -> TO_DCAN/89(ALM_DSCH_OCT_in)
  Rate Transition81/1 -> TO_DCAN/80(AMI_State_in)
  Rate Transition70/1 -> TO_DCAN/68(Point_MCU)
  Rate Transition97/1 -> TO_DCAN/96(ALM_BATT_UC_in)
  Rate Transition78/1 -> TO_DCAN/77(HV_Switch_in)
  Rate Transition88/1 -> TO_DCAN/87(ALM_HVREL_FAIL_in)
  Rate Transition96/1 -> TO_DCAN/95(ALM_BMU_FAIL_in)
  Rate Transition92/1 -> TO_DCAN/91(ALM_CHRG_OCT_in)
  Rate Transition56/1 -> TO_DCAN/54(Str_Over_SpdError_in)
  Rate Transition80/1 -> TO_DCAN/79(AS_Swtich_in)
  Rate Transition75/1 -> TO_DCAN/74(On_Out_Switch_in)
  Rate Transition71/1 -> TO_DCAN/69(Point_IPC)
  Rate Transition54/1 -> TO_DCAN/52(Str_Overvolt_Warning_in)
  Rate Transition60/1 -> TO_DCAN/58(Str_I2t_Warning_in)
  Rate Transition79/1 -> TO_DCAN/78(EBS_Rls_Switch_in)
  Rate Transition58/1 -> TO_DCAN/56(Swtiched_On_in)
  Rate Transition55/1 -> TO_DCAN/53(Str_Over_TopCurr_in)
  Rate Transition83/1 -> TO_DCAN/82(PosRlyStr_in)
  Rate Transition72/1 -> TO_DCAN/71(Point_BMS)
  Rate Transition74/1 -> TO_DCAN/73(Start_Swtich_in)
  Rate Transition76/1 -> TO_DCAN/75(On_In_Swtich_in)
  Rate Transition82/1 -> TO_DCAN/81(PreRlyStr_in)
  Rate Transition86/1 -> TO_DCAN/85(ALM_PRECHRG_FAIL_in)
  Rate Transition77/1 -> TO_DCAN/76(LV_Switch_in)
  Rate Transition89/1 -> TO_DCAN/88(ALM_HALL_BREAK_in)
  Rate Transition57/1 -> TO_DCAN/55(Str_Over_PosError_in)
  Rate Transition63/1 -> TO_DCAN/61(Str_Deg_in)
  Rate Transition108/1 -> TO_DCAN/107(ALM_CELL_UV_in)
  Rate Transition91/1 -> TO_DCAN/90(ALM_DSCH_OCS_in)
  Rate Transition94/1 -> TO_DCAN/93(ALM_BSU_OFFLINE_in)
  Rate Transition87/1 -> TO_DCAN/86(ALM_LEAK_OC_in)
  Rate Transition111/1 -> TO_DCAN/110(MaxTempNo_in)
  Rate Transition95/1 -> TO_DCAN/94(ALM_BSU_FAULT_in)
  Rate Transition106/1 -> TO_DCAN/105(ALM_CELL_UT_in)
  Rate Transition98/1 -> TO_DCAN/97(ALM_BATT_OC_in)
  Rate Transition100/1 -> TO_DCAN/99(ALM_BATT_UV_in)
  Rate Transition118/1 -> TO_DCAN/117(BatLife_in)
  Rate Transition121/1 -> TO_DCAN/120(BatSoh_in)
  Rate Transition116/1 -> TO_DCAN/115(MinCellVolt_in)
  Rate Transtion33/1 -> TO_DCAN/1(High_voltage_on)
  Rate Transition109/1 -> TO_DCAN/108(ALM_CELL_OV_in)
  Rate Transition114/1 -> TO_DCAN/113(MaxCellVoltNo_in)
  Rate Transition119/1 -> TO_DCAN/118(BatAlmLv_in)
  Rate Transition112/1 -> TO_DCAN/111(MinTemp_in)
  Rate Transition104/1 -> TO_DCAN/103(ALM_CELL_TBK_in)
  Rate Transition124/1 -> TO_DCAN/123(BatVoltage_in)
  Rate Transition107/1 -> TO_DCAN/106(ALM_CELL_OT_in)
  Rate Transition113/1 -> TO_DCAN/112(MaxTemp_in)
  Rate Transition115/1 -> TO_DCAN/114(MinCellVoltNo_in)
  Rate Transition120/1 -> TO_DCAN/119(BatState_in)
  Rate Transition123/1 -> TO_DCAN/122(BatCurrent_in)
  Rate Transition110/1 -> TO_DCAN/109(MinTempNo_in)
  Rate Transition101/1 -> TO_DCAN/100(ALM_BATT_OV_in)
  Rate Transition105/1 -> TO_DCAN/104(ALM_CELL_IBK_in)
  Rate Transition122/1 -> TO_DCAN/121(BatSoc_in)
  Rate Transition84/1 -> TO_DCAN/83(OnChrRlyStr_in)
  Rate Transition99/1 -> TO_DCAN/98(ALM_AUX_FAIL_in)
  Rate Transition103/1 -> TO_DCAN/102(ALM_BATT_DV_in)
  Rate Transition102/1 -> TO_DCAN/101(ALM_BATT_DT_in)
  Rate Transition117/1 -> TO_DCAN/116(MaxCellVolt_in)
  [FunCall_100ms_Duty1] -> TO_DCAN/Trigger
  TO_DCAN/1(DIAG_Bcu) -> Rate Transtion1/1
  TO_DCAN/2(DIAG_VEH_SENSOR) -> Rate Transtion2/1
  TO_DCAN/3(DIAG_WHL_Speed) -> Rate Transtion3/1
  TO_DCAN/4(DIAG_RES_DATA) -> Rate Transtion5/1
  TO_DCAN/5(DIAG_Scu) -> Rate Transtion6/1
  TO_DCAN/6(DIAG_VEH_INFO) -> Rate Transtion8/1
  TO_DCAN/7(DIAG_BMS_ALARM_RELAy) -> Rate Transtion9/1
  TO_DCAN/8(DIAG_BMS_MAXt) -> Rate Transtion10/1
  TO_DCAN/9(DIAG_BMS_MAXv) -> Rate Transtion11/1
  TO_DCAN/10(DIAG_BMS_INFo) -> Rate Transtion12/1
  Rate Transtion1/1 -> [DIAG_BCU_MESSAGE]
  Rate Transtion2/1 -> [DIAG_VEH_SENSOR]
  Rate Transtion3/1 -> [DIAG_WHL_SPD]
  Rate Transtion5/1 -> [DIAG_RES_Data_Message]
  Rate Transtion6/1 -> [DIAG_SCU_Message]
  Rate Transtion8/1 -> [DIAG_VEH_INFO]
  Rate Transtion9/1 -> [DIAG_BMS_ALARM_RELAY_Message]
  Rate Transtion10/1 -> [DIAG_BMS_MAXT_Message]
  Rate Transtion11/1 -> [DIAG_BMS_MAXV_Message]
  Rate Transtion12/1 -> [DIAG_BMS_INFO_Message]
  [Acc_Right_Disp_Val] -> Rate Transition6/1
  [Motor_Node] -> Rate Transition3/1
  Rate Transition3/1 -> TO_DCAN/70(Motor_Node)
  [Brk_Disp_Error] -> Rate Transition4/1
  Rate Transition4/1 -> TO_DCAN/129(Brk_Disp_SN_Sts)
  [Acc_Lft_Dip_Error] -> Rate Transition33/1
  Rate Transition33/1 -> TO_DCAN/130(Acc_Lft_Dip_Sts)
  [Acc_Right_Disp_Error] -> Rate Transition125/1
  Rate Transition125/1 -> TO_DCAN/131(Acc_Right_Dip_Sts)
  [BMS_Output_Volt_Error] -> Rate Transition126/1
  Rate Transition126/1 -> TO_DCAN/125(Volt_Cmp_BMS_Sts)
  [Mtr_Input_Volt_Error] -> Rate Transition127/1
  Rate Transition127/1 -> TO_DCAN/124(Volt_Cmp_Mtr_Sts)
  [Brs_Liq_Prs_Error] -> Rate Transition128/1
  Rate Transition128/1 -> TO_DCAN/126("Brs_Liq_Prs_Sts ")
  Rate Transition129/1 -> TO_DCAN/127(EBS_Gas_SN_2_Sts)
  Rate Transition130/1 -> TO_DCAN/128(EBS_Gas_SN_1_Sts)
  Rate Transtion131/1 -> TO_DCAN/4(AS_State)
  [EBS_GAP_pRS_2_Error] -> Rate Transition129/1
  [EBS_GAP_pRS_1_Error] -> Rate Transition130/1

== system FSAC2021_V1_Running/TASK_SCHEDULE ==
  Demux : Demux  Outputs=11
  Demux1 : Demux  Outputs=3
  Function-Call Generator : simulink/Ports & Subsystems/Function-Call Generator  sample_time=0.02  numberOfIterations=1
  Function-Call Generator1 : simulink/Ports & Subsystems/Function-Call Generator  sample_time=0.05  numberOfIterations=1
  Function-Call Generator2 : simulink/Ports & Subsystems/Function-Call Generator  sample_time=0.1  numberOfIterations=1
  Function-Call Generator3 : simulink/Ports & Subsystems/Function-Call Generator  sample_time=0.2  numberOfIterations=1
  tag scope: FunCall_100ms_Duty1=global, FunCall_100ms_Duty2=global, FunCall_100ms_Duty3=global, FunCall_200ms_Duty=global, FunCall_20ms_Duty=global, FunCall_50ms_Duty10=global, FunCall_50ms_Duty11=global, FunCall_50ms_Duty1=global, FunCall_50ms_Duty2=global, FunCall_50ms_Duty3=global, FunCall_50ms_Duty4=global, FunCall_50ms_Duty5=global, FunCall_50ms_Duty6=global, FunCall_50ms_Duty7=global, FunCall_50ms_Duty8=global, FunCall_50ms_Duty9=global
  wires:
  Function-Call Generator/1 -> [FunCall_20ms_Duty]
  Function-Call Generator1/1 -> Demux/1
  Demux/1 -> [FunCall_50ms_Duty1]
  Demux/2 -> [FunCall_50ms_Duty2]
  Demux/3 -> [FunCall_50ms_Duty3]
  Demux/5 -> [FunCall_50ms_Duty5]
  Demux/4 -> [FunCall_50ms_Duty4]
  Function-Call Generator2/1 -> Demux1/1
  Demux1/1 -> [FunCall_100ms_Duty1]
  Demux1/2 -> [FunCall_100ms_Duty2]
  Demux1/3 -> [FunCall_100ms_Duty3]
  Function-Call Generator3/1 -> [FunCall_200ms_Duty]
  Demux/6 -> [FunCall_50ms_Duty6]
  Demux/7 -> [FunCall_50ms_Duty7]
  Demux/8 -> [FunCall_50ms_Duty8]
  Demux/9 -> [FunCall_50ms_Duty9]
  Demux/10 -> [FunCall_50ms_Duty10]
  Demux/11 -> [FunCall_50ms_Duty11]
